simulink library "Lib_WindFilter"  (R2023a)
settings: Solver=VariableStepAuto  StartTime=0.0  StopTime=10.0  RelTol=1e-3
values from neighbouring files (symbols this model uses):
  wecs = 3.0    [DD_Mdl1.sldd]    (also in wecsmatfile.m = struct)
undefined symbols (not defined in the file or in its folder): DT, kVeFilt, kVeFilt_tau, step_thresshold
settings Model: Creator=ditt_aj  LastModifiedBy=ditt_aj

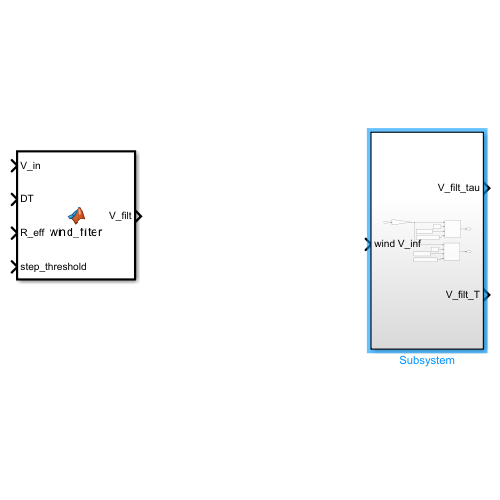
[thumbnail: Simulink's stored preview of the top-level diagram]
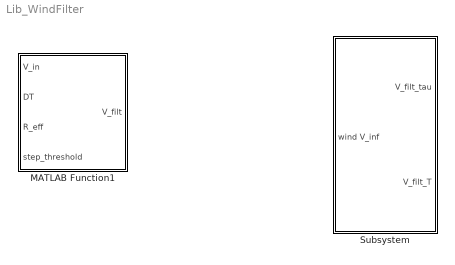
== system Lib_WindFilter ==
  MATLAB Function1 : MATLAB Function  TreatAsAtomicUnit=on
  Subsystem : Subsystem

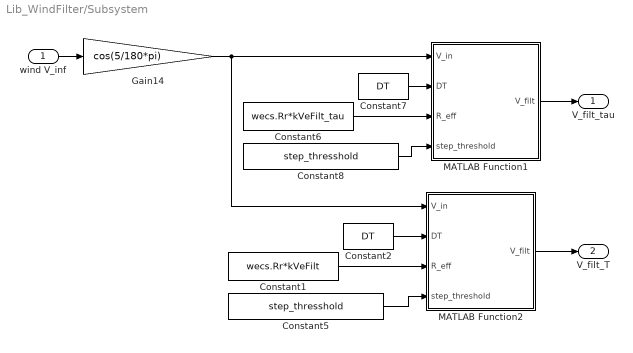
== system Lib_WindFilter/Subsystem ==
  wind V_inf : Inport
  Constant1 : Constant  Value=wecs.Rr*kVeFilt
  Constant2 : Constant  Value=DT
  Constant5 : Constant  Value=step_thresshold
  Constant6 : Constant  Value=wecs.Rr*kVeFilt_tau
  Constant7 : Constant  Value=DT
  Constant8 : Constant  Value=step_thresshold
  Gain14 : Gain  Gain=cos(5/180*pi)
  MATLAB Function1 : MATLAB Function  TreatAsAtomicUnit=on
  MATLAB Function2 : MATLAB Function  TreatAsAtomicUnit=on
  V_filt_tau : Outport
  V_filt_T : Outport  Port=2
  wires:
  Constant8/1 -> MATLAB Function1/4(step_threshold)
  Constant5/1 -> MATLAB Function2/4(step_threshold)
  Constant7/1 -> MATLAB Function1/2(DT)
  wind V_inf/1 -> Gain14/1
  Constant2/1 -> MATLAB Function2/2(DT)
  MATLAB Function2/1(V_filt) -> V_filt_T/1
  Constant6/1 -> MATLAB Function1/3(R_eff)
  Constant1/1 -> MATLAB Function2/3(R_eff)
  MATLAB Function1/1(V_filt) -> V_filt_tau/1
  Gain14/1 -> MATLAB Function2/1(V_in), MATLAB Function1/1(V_in)

== matlab function Lib_WindFilter/MATLAB Function1 ==
  settings: updateMethod=DISCRETE
  data: V_in input; V_filt output; DT input; R_eff input; step_threshold input
function V_filt = wind_filter(V_in, DT, R_eff,step_threshold)
% SPATIAL_WIND_FILTER 
% Implements a discrete, velocity-dependent low-pass filter for rotor-effective 
% wind speed estimation with an automated threshold bypass for step changes.

    % Persistent variables retain their state between time-steps
    persistent V_filt_prev V_in_prev 
    
    % --- Step 1: Handle Simulation Initialization ---
    if isempty( V_filt_prev) 
        V_filt_prev    = V_in; % Initialize filter state to current wind
        V_in_prev      = V_in; % Initialize raw input tracking
    end
    
    % --- Step 2: Compute Raw Wind Acceleration (Step Detection) ---
    % Calculate the true absolute sample-to-sample difference of the RAW wind
    delta_V_raw = abs(V_in - V_in_prev);
    
    % --- Step 3: Compute Filter Coefficient or Bypass ---
    % Compare with wind step threshold, e.g., 0.5 m/s jump between steps of 0.008s
    
    if delta_V_raw > step_threshold
        % If a non-physical step change is detected, snap alpha wide open
        alpha = 1.0;
    else
        %Otherwise, use the physical velocity-dependent spatial filter
        %Ensure V_in is bound to prevent division by zero at startup
        V_bound = max(V_in, 0.1); 
        alpha = 1.0 - exp(- (DT * V_bound) / R_eff);
        
       % Spherically bound alpha to normal discrete operational limits [0, 1]
        alpha = max(min(alpha, 1.0), 0.0);
   end
    
    % --- Step 4: Run the Filter Difference Equation ---
    V_filt = V_filt_prev + alpha * (V_in - V_filt_prev);
    
    % --- Step 5: Save State Registers for Next Step ---
    V_filt_prev = V_filt;
    V_in_prev   = V_in;
end

== matlab function Lib_WindFilter/Subsystem/MATLAB Function2 ==
  settings: updateMethod=DISCRETE
  data: V_in input; V_filt output; DT input; R_eff input; step_threshold input
function V_filt = wind_filter(V_in, DT, R_eff,step_threshold)
% SPATIAL_WIND_FILTER 
% Implements a discrete, velocity-dependent low-pass filter for rotor-effective 
% wind speed estimation with an automated threshold bypass for step changes.

    % Persistent variables retain their state between time-steps
    persistent V_filt_prev V_in_prev 
    
    % --- Step 1: Handle Simulation Initialization ---
    if isempty( V_filt_prev) 
        V_filt_prev    = V_in; % Initialize filter state to current wind
        V_in_prev      = V_in; % Initialize raw input tracking
    end
    
    % --- Step 2: Compute Raw Wind Acceleration (Step Detection) ---
    % Calculate the true absolute sample-to-sample difference of the RAW wind
    delta_V_raw = abs(V_in - V_in_prev);
    
    % --- Step 3: Compute Filter Coefficient or Bypass ---
    % Compare with wind step threshold, e.g., 0.5 m/s jump between steps of 0.008s
    
    if delta_V_raw > step_threshold
        % If a non-physical step change is detected, snap alpha wide open
        alpha = 1.0;
    else
        %Otherwise, use the physical velocity-dependent spatial filter
        %Ensure V_in is bound to prevent division by zero at startup
        V_bound = max(V_in, 0.1); 
        alpha = 1.0 - exp(- (DT * V_bound) / R_eff);
        
       % Spherically bound alpha to normal discrete operational limits [0, 1]
        alpha = max(min(alpha, 1.0), 0.0);
   end
    
    % --- Step 4: Run the Filter Difference Equation ---
    V_filt = V_filt_prev + alpha * (V_in - V_filt_prev);
    
    % --- Step 5: Save State Registers for Next Step ---
    V_filt_prev = V_filt;
    V_in_prev   = V_in;
end

== matlab function Lib_WindFilter/Subsystem/MATLAB Function1 ==
  settings: updateMethod=DISCRETE
  data: V_in input; V_filt output; DT input; R_eff input; step_threshold input
function V_filt = wind_filter(V_in, DT, R_eff,step_threshold)
% SPATIAL_WIND_FILTER 
% Implements a discrete, velocity-dependent low-pass filter for rotor-effective 
% wind speed estimation with an automated threshold bypass for step changes.

    % Persistent variables retain their state between time-steps
    persistent V_filt_prev V_in_prev 
    
    % --- Step 1: Handle Simulation Initialization ---
    if isempty( V_filt_prev) 
        V_filt_prev    = V_in; % Initialize filter state to current wind
        V_in_prev      = V_in; % Initialize raw input tracking
    end
    
    % --- Step 2: Compute Raw Wind Acceleration (Step Detection) ---
    % Calculate the true absolute sample-to-sample difference of the RAW wind
    delta_V_raw = abs(V_in - V_in_prev);
    
    % --- Step 3: Compute Filter Coefficient or Bypass ---
    % Compare with wind step threshold, e.g., 0.5 m/s jump between steps of 0.008s
    
    if delta_V_raw > step_threshold
        % If a non-physical step change is detected, snap alpha wide open
        alpha = 1.0;
    else
        %Otherwise, use the physical velocity-dependent spatial filter
        %Ensure V_in is bound to prevent division by zero at startup
        V_bound = max(V_in, 0.1); 
        alpha = 1.0 - exp(- (DT * V_bound) / R_eff);
        
       % Spherically bound alpha to normal discrete operational limits [0, 1]
        alpha = max(min(alpha, 1.0), 0.0);
   end
    
    % --- Step 4: Run the Filter Difference Equation ---
    V_filt = V_filt_prev + alpha * (V_in - V_filt_prev);
    
    % --- Step 5: Save State Registers for Next Step ---
    V_filt_prev = V_filt;
    V_in_prev   = V_in;
end
